simulink model "HMAUVSimulinkmobina"  (R2022b)
settings: Solver=ode45  StartTime=0.0  StopTime=80  MaxStep=0.01  RelTol=1e-3
libraries: slpidlib x6
settings Model: Creator=mobin  LastModifiedBy=mobin
settings SolverCC: AlgebraicLoopSolver=TrustRegion
settings DebuggingCC: UnconnectedInputMsg=warning  UnconnectedOutputMsg=warning  UnconnectedLineMsg=warning  SFMachineParentedDataDiag=warning
settings ModelReferenceCC: EnableRefExpFcnMdlSchedulingChecks=on
settings RTWCC: DLArmComputeVersion=19.05

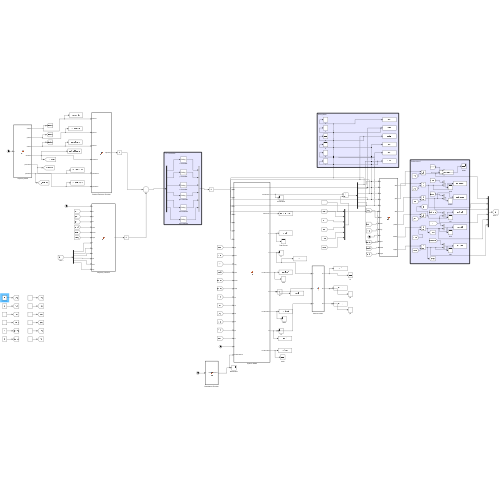
[thumbnail: Simulink's stored preview of the top-level diagram]
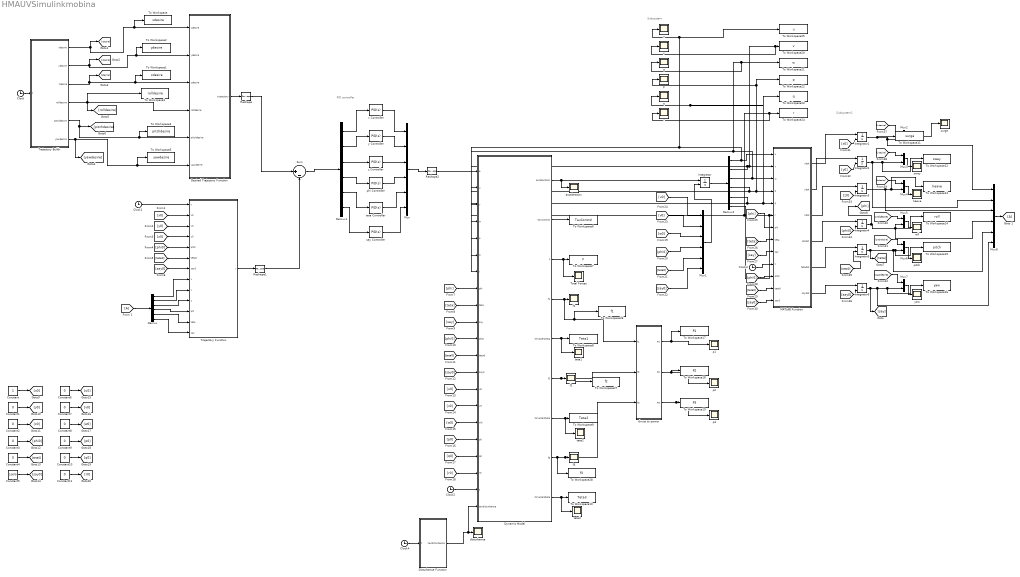
== system HMAUVSimulinkmobina ==
  note: Subsystem
  note: Subsystem1
  note: PID controller
  Clock{,1..4} (5 alike) : Clock
  Constant : Constant
  Constant{1..4,6..11} (10 alike) : Constant  Value=0
  Constant5 : Constant  Value=3.0079
  Demux : Demux  Outputs=6
  Demux1 : Demux  Outputs=6
  Demux2 : Demux  Outputs=6
  Desired Trajectory Function : MATLAB Function  TreatAsAtomicUnit=on
  Disturbance Function : MATLAB Function  TreatAsAtomicUnit=on
  Dynamic Model : MATLAB Function  TreatAsAtomicUnit=on
  From 1 : From
  Goto 1 : Goto
  Integrator{,1..6} (7 alike) : Integrator  InitialConditionSource=external
  MATLAB Function : MATLAB Function  TreatAsAtomicUnit=on
  Mux : Mux  Inputs=6
  Mux1 : Mux  Inputs=6
  Mux{2..7} (6 alike) : Mux  Inputs=2
  Mux8 : Mux  Inputs=6
  Reshape : Reshape  OutputDimensionality=Customize  OutputDimensions=[6,1]
  Reshape1 : Reshape  OutputDimensionality=Customize  OutputDimensions=[6,1]
  Reshape2 : Reshape  OutputDimensionality=Customize  OutputDimensions=[6,1]
  Sum : Sum  Inputs=|+-
  To Workspace : ToWorkspace  VariableName=xdesire  SaveFormat=Timeseries  SampleTime=-1
  To Workspace1 : ToWorkspace  VariableName=zdesire  SaveFormat=Timeseries  SampleTime=-1
  To Workspace10 : ToWorkspace  VariableName=Teta3  SaveFormat=Timeseries  SampleTime=-1
  To Workspace11 : ToWorkspace  VariableName=surge  SaveFormat=Timeseries  SampleTime=-1
  To Workspace12 : ToWorkspace  VariableName=sway  SaveFormat=Timeseries  SampleTime=-1
  To Workspace13 : ToWorkspace  VariableName=heave  SaveFormat=Timeseries  SampleTime=-1
  To Workspace14 : ToWorkspace  VariableName=roll  SaveFormat=Timeseries  SampleTime=-1
  To Workspace15 : ToWorkspace  VariableName=pitch  SaveFormat=Timeseries  SampleTime=-1
  To Workspace16 : ToWorkspace  VariableName=yaw  SaveFormat=Timeseries  SampleTime=-1
  To Workspace17 : ToWorkspace  VariableName=P1  SaveFormat=Timeseries  SampleTime=-1
  To Workspace18 : ToWorkspace  VariableName=P2  SaveFormat=Timeseries  SampleTime=-1
  To Workspace19 : ToWorkspace  VariableName=P3  SaveFormat=Timeseries  SampleTime=-1
  To Workspace2 : ToWorkspace  VariableName=ydesire  SaveFormat=Timeseries  SampleTime=-1
  To Workspace20 : ToWorkspace  VariableName=v  SaveFormat=Timeseries  SampleTime=-1
  To Workspace21 : ToWorkspace  VariableName=w  SaveFormat=Timeseries  SampleTime=-1
  To Workspace22 : ToWorkspace  VariableName=p  SaveFormat=Timeseries  SampleTime=-1
  To Workspace23 : ToWorkspace  VariableName=q  SaveFormat=Timeseries  SampleTime=-1
  To Workspace24 : ToWorkspace  VariableName=r  SaveFormat=Timeseries  SampleTime=-1
  To Workspace25 : ToWorkspace  VariableName=u  SaveFormat=Timeseries  SampleTime=-1
  To Workspace26 : ToWorkspace  VariableName=f1  SaveFormat=Timeseries  SampleTime=-1
  To Workspace27 : ToWorkspace  VariableName=f2  SaveFormat=Timeseries  SampleTime=-1
  To Workspace28 : ToWorkspace  VariableName=f3  SaveFormat=Timeseries  SampleTime=-1
  To Workspace3 : ToWorkspace  VariableName=rolldesire  SaveFormat=Timeseries  SampleTime=-1
  To Workspace4 : ToWorkspace  VariableName=pitchdesire  SaveFormat=Timeseries  SampleTime=-1
  To Workspace5 : ToWorkspace  VariableName=yawdesire  SaveFormat=Timeseries  SampleTime=-1
  To Workspace6 : ToWorkspace  VariableName=TavControl  SaveFormat=Timeseries  SampleTime=-1
  To Workspace7 : ToWorkspace  VariableName=F  SaveFormat=Timeseries  SampleTime=-1
  To Workspace8 : ToWorkspace  VariableName=Teta1  SaveFormat=Timeseries  SampleTime=-1
  To Workspace9 : ToWorkspace  VariableName=Teta2  SaveFormat=Timeseries  SampleTime=-1
  Total Forces : Scope
  Trajectory Buildr : MATLAB Function  TreatAsAtomicUnit=on
  Trajectory Function : MATLAB Function  TreatAsAtomicUnit=on
  acceleration : Scope
  disturbance : Scope
  f1 : Scope
  f2 : Scope
  f3 : Scope
  heave : Scope
  p{,1..3} (4 alike) : Scope
  phi Controller : slpidlib/PID Controller  Controller=PID  Form=Parallel  TimeDomain=Continuous-time  UseExternalTs=off  SampleTime=-1  IntegratorMethod=Forward Euler  FilterMethod=Forward Euler  ControllerParametersSource=internal  P=6000  I=0  UseKiTs=off  D=3000  N=100  UseFilter=on  TunerSelectOption=Transfer Function Based (PID Tuner App)  InitialConditionSource=internal  InitialConditionForIntegrator=0  InitialConditionForFilter=0  DifferentiatorICPrevScaledInput=0  ExternalReset=none  TrackingMode=off  Kt=1  LimitOutput=off  SatLimitsSource=internal  UpperSaturationLimit=inf  LowerSaturationLimit=-inf  LinearizeAsGain=on  AntiWindupMode=none  Kb=1  LimitIntegrator=off  UpperIntegratorSaturationLimit=inf  LowerIntegratorSaturationLimit=-inf  POutMin=[]  POutMax=[]  IOutMin=[]  IOutMax=[]  DOutMin=[]  DOutMax=[]  NOutMin=[]  NOutMax=[]  SumOutMin=[]  SumOutMax=[]  SaturationOutMin=[]  SaturationOutMax=[]  PParamMin=[]  PParamMax=[]  IParamMin=[]  IParamMax=[]  DParamMin=[]  DParamMax=[]  NParamMin=[]  NParamMax=[]  KbParamMin=[]  KbParamMax=[]  KtParamMin=[]  KtParamMax=[]  KbOutMin=[]  KbOutMax=[]  KtOutMin=[]  KtOutMax=[]  IntegratorOutMin=[]  IntegratorOutMax=[]  FilterOutMin=[]  FilterOutMax=[]  SumI1OutMin=[]  SumI1OutMax=[]  SumI2OutMin=[]  SumI2OutMax=[]  SumI3OutMin=[]  SumI3OutMax=[]  SumI4OutMin=[]  SumI4OutMax=[]  SumDOutMin=[]  SumDOutMax=[]  DifferentiatorOutMin=[]  DifferentiatorOutMax=[]  FilterDiffOutCoefMin=[]  FilterDiffOutCoefMax=[]  ReciprocalOutMin=[]  ReciprocalOutMax=[]  SumDenOutMin=[]  SumDenOutMax=[]  SumNumOutMin=[]  SumNumOutMax=[]  DivideOutMin=[]  DivideOutMax=[]  UdiffTsProdOutMin=[]  UdiffTsProdOutMax=[]  NTsProdOutMin=[]  NTsProdOutMax=[]  UintegralTsProdOutMin=[]  UintegralTsProdOutMax=[]  UngainTsProdOutMin=[]  UngainTsProdOutMax=[]  ClampingZeroOutDataTypeStr=Inherit: Inherit via back propagation  ClampingZeroOutMin=[]  ClampingZeroOutMax=[]  FilterDenConstantOutDataTypeStr=Inherit: Inherit via back propagation  FilterDenConstantOutMin=[]  FilterDenConstantOutMax=[]  PCopyOutDataTypeStr=Inherit: Inherit via back propagation  PCopyOutMin=[]  PCopyOutMax=[]  NCopyOutDataTypeStr=Inherit: Inherit via back propagation  NCopyOutMin=[]  NCopyOutMax=[]  IntegratorContinuousStateAttributes=''  IntegratorStateMustResolveToSignalObject=off  IntegratorRTWStateStorageClass=Auto  FilterContinuousStateAttributes=''  FilterStateMustResolveToSignalObject=off  FilterRTWStateStorageClass=Auto  ParallelPVariant=InternalParameters  IdealPVariant=Disabled  IVariant=InternalParameters  DVariant=InternalParameters  IntegratorVariant=Continuous  SatVariant=Disabled  AWVariant=Passthrough  PCopyVariant=Disabled  TRVariant=Disabled  FdbkBlocksVariant=Forward  IdealPFdbkVariant=Disabled  SatFdbkVariant=Disabled  DerivativeFilterVariant=ContFilter  NVariant=InternalParameters  NCopyVariant=Disabled  FilterICVariant=InternalICsFilter  IntegratorICVariant=InternalICs  ExternalResetVariant=Disabled  TRSumVariant=Passthrough  SumFdbkVariant=Disabled  SumVariant=Sum_PID  TsampFilterVariant=InternalTs  TsampNgainVariant=Passthrough  TsampIntegralVariant=Passthrough  ExternalSaturationOutDataTypeStr=Inherit: Same as second input
  pitch : Scope
  q : Scope
  r : Scope
  roll : Scope
  say Controller : slpidlib/PID Controller  Controller=PID  Form=Parallel  TimeDomain=Continuous-time  UseExternalTs=off  SampleTime=-1  IntegratorMethod=Forward Euler  FilterMethod=Forward Euler  ControllerParametersSource=internal  P=6000  I=0  UseKiTs=off  D=3000  N=100  UseFilter=on  TunerSelectOption=Transfer Function Based (PID Tuner App)  InitialConditionSource=internal  InitialConditionForIntegrator=0  InitialConditionForFilter=0  DifferentiatorICPrevScaledInput=0  ExternalReset=none  TrackingMode=off  Kt=1  LimitOutput=off  SatLimitsSource=internal  UpperSaturationLimit=inf  LowerSaturationLimit=-inf  LinearizeAsGain=on  AntiWindupMode=none  Kb=1  LimitIntegrator=off  UpperIntegratorSaturationLimit=inf  LowerIntegratorSaturationLimit=-inf  POutMin=[]  POutMax=[]  IOutMin=[]  IOutMax=[]  DOutMin=[]  DOutMax=[]  NOutMin=[]  NOutMax=[]  SumOutMin=[]  SumOutMax=[]  SaturationOutMin=[]  SaturationOutMax=[]  PParamMin=[]  PParamMax=[]  IParamMin=[]  IParamMax=[]  DParamMin=[]  DParamMax=[]  NParamMin=[]  NParamMax=[]  KbParamMin=[]  KbParamMax=[]  KtParamMin=[]  KtParamMax=[]  KbOutMin=[]  KbOutMax=[]  KtOutMin=[]  KtOutMax=[]  IntegratorOutMin=[]  IntegratorOutMax=[]  FilterOutMin=[]  FilterOutMax=[]  SumI1OutMin=[]  SumI1OutMax=[]  SumI2OutMin=[]  SumI2OutMax=[]  SumI3OutMin=[]  SumI3OutMax=[]  SumI4OutMin=[]  SumI4OutMax=[]  SumDOutMin=[]  SumDOutMax=[]  DifferentiatorOutMin=[]  DifferentiatorOutMax=[]  FilterDiffOutCoefMin=[]  FilterDiffOutCoefMax=[]  ReciprocalOutMin=[]  ReciprocalOutMax=[]  SumDenOutMin=[]  SumDenOutMax=[]  SumNumOutMin=[]  SumNumOutMax=[]  DivideOutMin=[]  DivideOutMax=[]  UdiffTsProdOutMin=[]  UdiffTsProdOutMax=[]  NTsProdOutMin=[]  NTsProdOutMax=[]  UintegralTsProdOutMin=[]  UintegralTsProdOutMax=[]  UngainTsProdOutMin=[]  UngainTsProdOutMax=[]  ClampingZeroOutDataTypeStr=Inherit: Inherit via back propagation  ClampingZeroOutMin=[]  ClampingZeroOutMax=[]  FilterDenConstantOutDataTypeStr=Inherit: Inherit via back propagation  FilterDenConstantOutMin=[]  FilterDenConstantOutMax=[]  PCopyOutDataTypeStr=Inherit: Inherit via back propagation  PCopyOutMin=[]  PCopyOutMax=[]  NCopyOutDataTypeStr=Inherit: Inherit via back propagation  NCopyOutMin=[]  NCopyOutMax=[]  IntegratorContinuousStateAttributes=''  IntegratorStateMustResolveToSignalObject=off  IntegratorRTWStateStorageClass=Auto  FilterContinuousStateAttributes=''  FilterStateMustResolveToSignalObject=off  FilterRTWStateStorageClass=Auto  ParallelPVariant=InternalParameters  IdealPVariant=Disabled  IVariant=InternalParameters  DVariant=InternalParameters  IntegratorVariant=Continuous  SatVariant=Disabled  AWVariant=Passthrough  PCopyVariant=Disabled  TRVariant=Disabled  FdbkBlocksVariant=Forward  IdealPFdbkVariant=Disabled  SatFdbkVariant=Disabled  DerivativeFilterVariant=ContFilter  NVariant=InternalParameters  NCopyVariant=Disabled  FilterICVariant=InternalICsFilter  IntegratorICVariant=InternalICs  ExternalResetVariant=Disabled  TRSumVariant=Passthrough  SumFdbkVariant=Disabled  SumVariant=Sum_PID  TsampFilterVariant=InternalTs  TsampNgainVariant=Passthrough  TsampIntegralVariant=Passthrough  ExternalSaturationOutDataTypeStr=Inherit: Same as second input
  surge : Scope
  sway : Scope
  teta Controller : slpidlib/PID Controller  Controller=PID  Form=Parallel  TimeDomain=Continuous-time  UseExternalTs=off  SampleTime=-1  IntegratorMethod=Forward Euler  FilterMethod=Forward Euler  ControllerParametersSource=internal  P=6000  I=0  UseKiTs=off  D=3000  N=100  UseFilter=on  TunerSelectOption=Transfer Function Based (PID Tuner App)  InitialConditionSource=internal  InitialConditionForIntegrator=0  InitialConditionForFilter=0  DifferentiatorICPrevScaledInput=0  ExternalReset=none  TrackingMode=off  Kt=1  LimitOutput=off  SatLimitsSource=internal  UpperSaturationLimit=inf  LowerSaturationLimit=-inf  LinearizeAsGain=on  AntiWindupMode=none  Kb=1  LimitIntegrator=off  UpperIntegratorSaturationLimit=inf  LowerIntegratorSaturationLimit=-inf  POutMin=[]  POutMax=[]  IOutMin=[]  IOutMax=[]  DOutMin=[]  DOutMax=[]  NOutMin=[]  NOutMax=[]  SumOutMin=[]  SumOutMax=[]  SaturationOutMin=[]  SaturationOutMax=[]  PParamMin=[]  PParamMax=[]  IParamMin=[]  IParamMax=[]  DParamMin=[]  DParamMax=[]  NParamMin=[]  NParamMax=[]  KbParamMin=[]  KbParamMax=[]  KtParamMin=[]  KtParamMax=[]  KbOutMin=[]  KbOutMax=[]  KtOutMin=[]  KtOutMax=[]  IntegratorOutMin=[]  IntegratorOutMax=[]  FilterOutMin=[]  FilterOutMax=[]  SumI1OutMin=[]  SumI1OutMax=[]  SumI2OutMin=[]  SumI2OutMax=[]  SumI3OutMin=[]  SumI3OutMax=[]  SumI4OutMin=[]  SumI4OutMax=[]  SumDOutMin=[]  SumDOutMax=[]  DifferentiatorOutMin=[]  DifferentiatorOutMax=[]  FilterDiffOutCoefMin=[]  FilterDiffOutCoefMax=[]  ReciprocalOutMin=[]  ReciprocalOutMax=[]  SumDenOutMin=[]  SumDenOutMax=[]  SumNumOutMin=[]  SumNumOutMax=[]  DivideOutMin=[]  DivideOutMax=[]  UdiffTsProdOutMin=[]  UdiffTsProdOutMax=[]  NTsProdOutMin=[]  NTsProdOutMax=[]  UintegralTsProdOutMin=[]  UintegralTsProdOutMax=[]  UngainTsProdOutMin=[]  UngainTsProdOutMax=[]  ClampingZeroOutDataTypeStr=Inherit: Inherit via back propagation  ClampingZeroOutMin=[]  ClampingZeroOutMax=[]  FilterDenConstantOutDataTypeStr=Inherit: Inherit via back propagation  FilterDenConstantOutMin=[]  FilterDenConstantOutMax=[]  PCopyOutDataTypeStr=Inherit: Inherit via back propagation  PCopyOutMin=[]  PCopyOutMax=[]  NCopyOutDataTypeStr=Inherit: Inherit via back propagation  NCopyOutMin=[]  NCopyOutMax=[]  IntegratorContinuousStateAttributes=''  IntegratorStateMustResolveToSignalObject=off  IntegratorRTWStateStorageClass=Auto  FilterContinuousStateAttributes=''  FilterStateMustResolveToSignalObject=off  FilterRTWStateStorageClass=Auto  ParallelPVariant=InternalParameters  IdealPVariant=Disabled  IVariant=InternalParameters  DVariant=InternalParameters  IntegratorVariant=Continuous  SatVariant=Disabled  AWVariant=Passthrough  PCopyVariant=Disabled  TRVariant=Disabled  FdbkBlocksVariant=Forward  IdealPFdbkVariant=Disabled  SatFdbkVariant=Disabled  DerivativeFilterVariant=ContFilter  NVariant=InternalParameters  NCopyVariant=Disabled  FilterICVariant=InternalICsFilter  IntegratorICVariant=InternalICs  ExternalResetVariant=Disabled  TRSumVariant=Passthrough  SumFdbkVariant=Disabled  SumVariant=Sum_PID  TsampFilterVariant=InternalTs  TsampNgainVariant=Passthrough  TsampIntegralVariant=Passthrough  ExternalSaturationOutDataTypeStr=Inherit: Same as second input
  teta1 : Scope
  teta2 : Scope
  teta3 : Scope
  thrust to power : MATLAB Function  TreatAsAtomicUnit=on
  u : Scope
  v : Scope
  w : Scope
  x Controller : slpidlib/PID Controller  Controller=PID  Form=Parallel  TimeDomain=Continuous-time  UseExternalTs=off  SampleTime=-1  IntegratorMethod=Forward Euler  FilterMethod=Forward Euler  ControllerParametersSource=internal  P=6000  I=0  UseKiTs=off  D=3000  N=100  UseFilter=on  TunerSelectOption=Transfer Function Based (PID Tuner App)  InitialConditionSource=internal  InitialConditionForIntegrator=0  InitialConditionForFilter=0  DifferentiatorICPrevScaledInput=0  ExternalReset=none  TrackingMode=off  Kt=1  LimitOutput=off  SatLimitsSource=internal  UpperSaturationLimit=inf  LowerSaturationLimit=-inf  LinearizeAsGain=on  AntiWindupMode=none  Kb=1  LimitIntegrator=off  UpperIntegratorSaturationLimit=inf  LowerIntegratorSaturationLimit=-inf  POutMin=[]  POutMax=[]  IOutMin=[]  IOutMax=[]  DOutMin=[]  DOutMax=[]  NOutMin=[]  NOutMax=[]  SumOutMin=[]  SumOutMax=[]  SaturationOutMin=[]  SaturationOutMax=[]  PParamMin=[]  PParamMax=[]  IParamMin=[]  IParamMax=[]  DParamMin=[]  DParamMax=[]  NParamMin=[]  NParamMax=[]  KbParamMin=[]  KbParamMax=[]  KtParamMin=[]  KtParamMax=[]  KbOutMin=[]  KbOutMax=[]  KtOutMin=[]  KtOutMax=[]  IntegratorOutMin=[]  IntegratorOutMax=[]  FilterOutMin=[]  FilterOutMax=[]  SumI1OutMin=[]  SumI1OutMax=[]  SumI2OutMin=[]  SumI2OutMax=[]  SumI3OutMin=[]  SumI3OutMax=[]  SumI4OutMin=[]  SumI4OutMax=[]  SumDOutMin=[]  SumDOutMax=[]  DifferentiatorOutMin=[]  DifferentiatorOutMax=[]  FilterDiffOutCoefMin=[]  FilterDiffOutCoefMax=[]  ReciprocalOutMin=[]  ReciprocalOutMax=[]  SumDenOutMin=[]  SumDenOutMax=[]  SumNumOutMin=[]  SumNumOutMax=[]  DivideOutMin=[]  DivideOutMax=[]  UdiffTsProdOutMin=[]  UdiffTsProdOutMax=[]  NTsProdOutMin=[]  NTsProdOutMax=[]  UintegralTsProdOutMin=[]  UintegralTsProdOutMax=[]  UngainTsProdOutMin=[]  UngainTsProdOutMax=[]  ClampingZeroOutDataTypeStr=Inherit: Inherit via back propagation  ClampingZeroOutMin=[]  ClampingZeroOutMax=[]  FilterDenConstantOutDataTypeStr=Inherit: Inherit via back propagation  FilterDenConstantOutMin=[]  FilterDenConstantOutMax=[]  PCopyOutDataTypeStr=Inherit: Inherit via back propagation  PCopyOutMin=[]  PCopyOutMax=[]  NCopyOutDataTypeStr=Inherit: Inherit via back propagation  NCopyOutMin=[]  NCopyOutMax=[]  IntegratorContinuousStateAttributes=''  IntegratorStateMustResolveToSignalObject=off  IntegratorRTWStateStorageClass=Auto  FilterContinuousStateAttributes=''  FilterStateMustResolveToSignalObject=off  FilterRTWStateStorageClass=Auto  ParallelPVariant=InternalParameters  IdealPVariant=Disabled  IVariant=InternalParameters  DVariant=InternalParameters  IntegratorVariant=Continuous  SatVariant=Disabled  AWVariant=Passthrough  PCopyVariant=Disabled  TRVariant=Disabled  FdbkBlocksVariant=Forward  IdealPFdbkVariant=Disabled  SatFdbkVariant=Disabled  DerivativeFilterVariant=ContFilter  NVariant=InternalParameters  NCopyVariant=Disabled  FilterICVariant=InternalICsFilter  IntegratorICVariant=InternalICs  ExternalResetVariant=Disabled  TRSumVariant=Passthrough  SumFdbkVariant=Disabled  SumVariant=Sum_PID  TsampFilterVariant=InternalTs  TsampNgainVariant=Passthrough  TsampIntegralVariant=Passthrough  ExternalSaturationOutDataTypeStr=Inherit: Same as second input
  y Controller : slpidlib/PID Controller  Controller=PID  Form=Parallel  TimeDomain=Continuous-time  UseExternalTs=off  SampleTime=-1  IntegratorMethod=Forward Euler  FilterMethod=Forward Euler  ControllerParametersSource=internal  P=6000  I=0  UseKiTs=off  D=3000  N=100  UseFilter=on  TunerSelectOption=Transfer Function Based (PID Tuner App)  InitialConditionSource=internal  InitialConditionForIntegrator=0  InitialConditionForFilter=0  DifferentiatorICPrevScaledInput=0  ExternalReset=none  TrackingMode=off  Kt=1  LimitOutput=off  SatLimitsSource=internal  UpperSaturationLimit=inf  LowerSaturationLimit=-inf  LinearizeAsGain=on  AntiWindupMode=none  Kb=1  LimitIntegrator=off  UpperIntegratorSaturationLimit=inf  LowerIntegratorSaturationLimit=-inf  POutMin=[]  POutMax=[]  IOutMin=[]  IOutMax=[]  DOutMin=[]  DOutMax=[]  NOutMin=[]  NOutMax=[]  SumOutMin=[]  SumOutMax=[]  SaturationOutMin=[]  SaturationOutMax=[]  PParamMin=[]  PParamMax=[]  IParamMin=[]  IParamMax=[]  DParamMin=[]  DParamMax=[]  NParamMin=[]  NParamMax=[]  KbParamMin=[]  KbParamMax=[]  KtParamMin=[]  KtParamMax=[]  KbOutMin=[]  KbOutMax=[]  KtOutMin=[]  KtOutMax=[]  IntegratorOutMin=[]  IntegratorOutMax=[]  FilterOutMin=[]  FilterOutMax=[]  SumI1OutMin=[]  SumI1OutMax=[]  SumI2OutMin=[]  SumI2OutMax=[]  SumI3OutMin=[]  SumI3OutMax=[]  SumI4OutMin=[]  SumI4OutMax=[]  SumDOutMin=[]  SumDOutMax=[]  DifferentiatorOutMin=[]  DifferentiatorOutMax=[]  FilterDiffOutCoefMin=[]  FilterDiffOutCoefMax=[]  ReciprocalOutMin=[]  ReciprocalOutMax=[]  SumDenOutMin=[]  SumDenOutMax=[]  SumNumOutMin=[]  SumNumOutMax=[]  DivideOutMin=[]  DivideOutMax=[]  UdiffTsProdOutMin=[]  UdiffTsProdOutMax=[]  NTsProdOutMin=[]  NTsProdOutMax=[]  UintegralTsProdOutMin=[]  UintegralTsProdOutMax=[]  UngainTsProdOutMin=[]  UngainTsProdOutMax=[]  ClampingZeroOutDataTypeStr=Inherit: Inherit via back propagation  ClampingZeroOutMin=[]  ClampingZeroOutMax=[]  FilterDenConstantOutDataTypeStr=Inherit: Inherit via back propagation  FilterDenConstantOutMin=[]  FilterDenConstantOutMax=[]  PCopyOutDataTypeStr=Inherit: Inherit via back propagation  PCopyOutMin=[]  PCopyOutMax=[]  NCopyOutDataTypeStr=Inherit: Inherit via back propagation  NCopyOutMin=[]  NCopyOutMax=[]  IntegratorContinuousStateAttributes=''  IntegratorStateMustResolveToSignalObject=off  IntegratorRTWStateStorageClass=Auto  FilterContinuousStateAttributes=''  FilterStateMustResolveToSignalObject=off  FilterRTWStateStorageClass=Auto  ParallelPVariant=InternalParameters  IdealPVariant=Disabled  IVariant=InternalParameters  DVariant=InternalParameters  IntegratorVariant=Continuous  SatVariant=Disabled  AWVariant=Passthrough  PCopyVariant=Disabled  TRVariant=Disabled  FdbkBlocksVariant=Forward  IdealPFdbkVariant=Disabled  SatFdbkVariant=Disabled  DerivativeFilterVariant=ContFilter  NVariant=InternalParameters  NCopyVariant=Disabled  FilterICVariant=InternalICsFilter  IntegratorICVariant=InternalICs  ExternalResetVariant=Disabled  TRSumVariant=Passthrough  SumFdbkVariant=Disabled  SumVariant=Sum_PID  TsampFilterVariant=InternalTs  TsampNgainVariant=Passthrough  TsampIntegralVariant=Passthrough  ExternalSaturationOutDataTypeStr=Inherit: Same as second input
  yaw : Scope
  z Controller : slpidlib/PID Controller  Controller=PID  Form=Parallel  TimeDomain=Continuous-time  UseExternalTs=off  SampleTime=-1  IntegratorMethod=Forward Euler  FilterMethod=Forward Euler  ControllerParametersSource=internal  P=6000  I=0  UseKiTs=off  D=3000  N=100  UseFilter=on  TunerSelectOption=Transfer Function Based (PID Tuner App)  InitialConditionSource=internal  InitialConditionForIntegrator=0  InitialConditionForFilter=0  DifferentiatorICPrevScaledInput=0  ExternalReset=none  TrackingMode=off  Kt=1  LimitOutput=off  SatLimitsSource=internal  UpperSaturationLimit=inf  LowerSaturationLimit=-inf  LinearizeAsGain=on  AntiWindupMode=none  Kb=1  LimitIntegrator=off  UpperIntegratorSaturationLimit=inf  LowerIntegratorSaturationLimit=-inf  POutMin=[]  POutMax=[]  IOutMin=[]  IOutMax=[]  DOutMin=[]  DOutMax=[]  NOutMin=[]  NOutMax=[]  SumOutMin=[]  SumOutMax=[]  SaturationOutMin=[]  SaturationOutMax=[]  PParamMin=[]  PParamMax=[]  IParamMin=[]  IParamMax=[]  DParamMin=[]  DParamMax=[]  NParamMin=[]  NParamMax=[]  KbParamMin=[]  KbParamMax=[]  KtParamMin=[]  KtParamMax=[]  KbOutMin=[]  KbOutMax=[]  KtOutMin=[]  KtOutMax=[]  IntegratorOutMin=[]  IntegratorOutMax=[]  FilterOutMin=[]  FilterOutMax=[]  SumI1OutMin=[]  SumI1OutMax=[]  SumI2OutMin=[]  SumI2OutMax=[]  SumI3OutMin=[]  SumI3OutMax=[]  SumI4OutMin=[]  SumI4OutMax=[]  SumDOutMin=[]  SumDOutMax=[]  DifferentiatorOutMin=[]  DifferentiatorOutMax=[]  FilterDiffOutCoefMin=[]  FilterDiffOutCoefMax=[]  ReciprocalOutMin=[]  ReciprocalOutMax=[]  SumDenOutMin=[]  SumDenOutMax=[]  SumNumOutMin=[]  SumNumOutMax=[]  DivideOutMin=[]  DivideOutMax=[]  UdiffTsProdOutMin=[]  UdiffTsProdOutMax=[]  NTsProdOutMin=[]  NTsProdOutMax=[]  UintegralTsProdOutMin=[]  UintegralTsProdOutMax=[]  UngainTsProdOutMin=[]  UngainTsProdOutMax=[]  ClampingZeroOutDataTypeStr=Inherit: Inherit via back propagation  ClampingZeroOutMin=[]  ClampingZeroOutMax=[]  FilterDenConstantOutDataTypeStr=Inherit: Inherit via back propagation  FilterDenConstantOutMin=[]  FilterDenConstantOutMax=[]  PCopyOutDataTypeStr=Inherit: Inherit via back propagation  PCopyOutMin=[]  PCopyOutMax=[]  NCopyOutDataTypeStr=Inherit: Inherit via back propagation  NCopyOutMin=[]  NCopyOutMax=[]  IntegratorContinuousStateAttributes=''  IntegratorStateMustResolveToSignalObject=off  IntegratorRTWStateStorageClass=Auto  FilterContinuousStateAttributes=''  FilterStateMustResolveToSignalObject=off  FilterRTWStateStorageClass=Auto  ParallelPVariant=InternalParameters  IdealPVariant=Disabled  IVariant=InternalParameters  DVariant=InternalParameters  IntegratorVariant=Continuous  SatVariant=Disabled  AWVariant=Passthrough  PCopyVariant=Disabled  TRVariant=Disabled  FdbkBlocksVariant=Forward  IdealPFdbkVariant=Disabled  SatFdbkVariant=Disabled  DerivativeFilterVariant=ContFilter  NVariant=InternalParameters  NCopyVariant=Disabled  FilterICVariant=InternalICsFilter  IntegratorICVariant=InternalICs  ExternalResetVariant=Disabled  TRSumVariant=Passthrough  SumFdbkVariant=Disabled  SumVariant=Sum_PID  TsampFilterVariant=InternalTs  TsampNgainVariant=Passthrough  TsampIntegralVariant=Passthrough  ExternalSaturationOutDataTypeStr=Inherit: Same as second input
  wires:
  Clock/1 -> Trajectory Buildr/1(t)
  Trajectory Buildr/1(xdesire) -> To Workspace/1, Desired Trajectory Function/1(xdesire), [xdesire]
  Trajectory Buildr/2(ydesire) -> To Workspace2/1, Desired Trajectory Function/2(ydesire), [ydesire]
  Trajectory Buildr/3(zdesire) -> [zdesire], To Workspace1/1, Desired Trajectory Function/3(zdesire)
  Clock1/1 -> Trajectory Function/1(t)
  Demux/1 -> Trajectory Function/8(x)
  Demux/2 -> Trajectory Function/9(y)
  Demux/3 -> Trajectory Function/10(z)
  Demux/4 -> Trajectory Function/11(phi)
  Demux/5 -> Trajectory Function/12(teta)
  Demux/6 -> Trajectory Function/13(say)
  From 1/1 -> Demux/1
  [x0] -> Trajectory Function/2(x0)
  [y0] -> Trajectory Function/3(y0)
  [z0] -> Trajectory Function/4(z0)
  [phi0] -> Trajectory Function/5(phi0)
  [teta0] -> Trajectory Function/6(teta0)
  [say0] -> Trajectory Function/7(say0)
  Trajectory Function/1(r) -> Reshape1/1
  Desired Trajectory Function/1(trajectory) -> Reshape/1
  [phi] -> Dynamic Model/8(phi)
  [teta] -> Dynamic Model/9(teta)
  [say] -> Dynamic Model/10(say)
  [phi0] -> Dynamic Model/11(phi0)
  [teta0] -> Dynamic Model/12(teta0)
  [say0] -> Dynamic Model/13(say0)
  [u0] -> Dynamic Model/14(u0)
  [v0] -> Dynamic Model/15(v0)
  [w0] -> Dynamic Model/16(w0)
  [p0] -> Dynamic Model/17(p0)
  [q0] -> Dynamic Model/18(q0)
  [r0] -> Dynamic Model/19(r0)
  Clock2/1 -> Dynamic Model/20(t)
  Dynamic Model/3(F) -> Total Forces/1, To Workspace7/1
  Dynamic Model/5(thruster1teta) -> teta1/1, To Workspace8/1
  Dynamic Model/7(thruster2teta) -> teta2/1, To Workspace9/1
  Dynamic Model/9(thruster3teta) -> teta3/1, To Workspace10/1
  Dynamic Model/4(f1) -> To Workspace26/1, thrust to power/1(f1), f1/1
  Dynamic Model/6(f2) -> To Workspace27/1, thrust to power/2(f2), f2/1
  Dynamic Model/8(f3) -> To Workspace28/1, thrust to power/3(f3), f3/1
  [u0] -> Mux1/1
  [v0] -> Mux1/2
  [w0] -> Mux1/3
  [phi0] -> Mux1/4
  [teta0] -> Mux1/5
  [say0] -> Mux1/6
  Mux1/1 -> Integrator/2
  Dynamic Model/1(accelaration) -> acceleration/1, Integrator/1
  Integrator/1 -> Demux2/1
  [phi] -> MATLAB Function/7(phi)
  [teta] -> MATLAB Function/8(teta)
  [say] -> MATLAB Function/9(say)
  [phi0] -> MATLAB Function/11(phi0)
  [teta0] -> MATLAB Function/12(teta0)
  [say0] -> MATLAB Function/13(say0)
  Clock3/1 -> MATLAB Function/10(t)
  Mux8/1 -> Goto 1/1
  thrust to power/1(P1) -> p1/1, To Workspace17/1
  thrust to power/2(P2) -> To Workspace18/1, p2/1
  thrust to power/3(P3) -> p3/1, To Workspace19/1
  Reshape/1 -> Sum/1
  Reshape1/1 -> Sum/2
  Constant/1 -> [x0]
  Constant1/1 -> [y0]
  Constant2/1 -> [z0]
  Constant3/1 -> [phi0]
  Constant4/1 -> [teta0]
  Constant5/1 -> [say0]
  Constant6/1 -> [u0]
  Constant7/1 -> [v0]
  Constant8/1 -> [w0]
  Constant9/1 -> [p0]
  Constant10/1 -> [q0]
  Constant11/1 -> [r0]
  Clock4/1 -> Disturbance Function/1(t)
  Disturbance Function/1(tavdisturbance) -> Dynamic Model/21(tavdisturbance), disturbance/1
  Reshape2/1 -> Dynamic Model/1(e)
  Mux/1 -> Reshape2/1
  Trajectory Buildr/4(rolldesire) -> Desired Trajectory Function/4(rolldesire), To Workspace3/1, [rolldesire]
  Trajectory Buildr/5(pitchdesire) -> [pitchdesire], To Workspace4/1, Desired Trajectory Function/5(pitchdesire)
  Trajectory Buildr/6(yawdesire) -> [yawdesire], To Workspace5/1, Desired Trajectory Function/6(yawdesire)
  Dynamic Model/2(TAVcontrol) -> To Workspace6/1
  Sum/1 -> Demux1/1
  phi Controller/1 -> Mux/4
  y Controller/1 -> Mux/2
  Demux1/3 -> z Controller/1
  Demux1/5 -> teta Controller/1
  x Controller/1 -> Mux/1
  Demux1/6 -> say Controller/1
  z Controller/1 -> Mux/3
  Demux1/1 -> x Controller/1
  Demux1/4 -> phi Controller/1
  say Controller/1 -> Mux/6
  Demux1/2 -> y Controller/1
  teta Controller/1 -> Mux/5
  Integrator1/1 -> To Workspace11/1, Mux8/1, Mux2/2
  Integrator2/1 -> Mux8/2, To Workspace12/1, Mux3/2
  Integrator3/1 -> Mux8/3, To Workspace13/1, Mux4/2
  Integrator4/1 -> [phi], Mux5/2, Mux8/4, To Workspace14/1
  Integrator5/1 -> [teta], Mux8/5, To Workspace15/1, Mux6/2
  Integrator6/1 -> [say], Mux8/6, To Workspace16/1, Mux7/2
  MATLAB Function/3(zdot) -> Integrator3/1
  MATLAB Function/6(saydot) -> Integrator6/1
  [xdesire] -> Mux2/1
  Mux5/1 -> roll/1
  Mux6/1 -> pitch/1
  MATLAB Function/4(phidot) -> Integrator4/1
  Mux2/1 -> surge/1
  MATLAB Function/1(xdot) -> Integrator1/1
  Mux3/1 -> sway/1
  MATLAB Function/5(tetadot) -> Integrator5/1
  Mux7/1 -> yaw/1
  [yawdesire] -> Mux7/1
  [phi0] -> Integrator4/2
  [pitchdesire] -> Mux6/1
  [say0] -> Integrator6/2
  [rolldesire] -> Mux5/1
  [ydesire] -> Mux3/1
  [y0] -> Integrator2/2
  Mux4/1 -> heave/1
  [teta0] -> Integrator5/2
  [z0] -> Integrator3/2
  [x0] -> Integrator1/2
  MATLAB Function/2(ydot) -> Integrator2/1
  [zdesire] -> Mux4/1
  Demux2/3 -> Dynamic Model/4(w), w/1, To Workspace21/1, MATLAB Function/3(w)
  Demux2/4 -> To Workspace22/1, p/1, MATLAB Function/4(p), Dynamic Model/5(p)
  Demux2/5 -> MATLAB Function/5(q), To Workspace23/1, q/1, Dynamic Model/6(q)
  Demux2/1 -> MATLAB Function/1(u), Dynamic Model/2(u), To Workspace25/1, u/1
  Demux2/6 -> r/1, To Workspace24/1, Dynamic Model/7(r), MATLAB Function/6(r)
  Demux2/2 -> v/1, To Workspace20/1, MATLAB Function/2(v), Dynamic Model/3(v)

== matlab function HMAUVSimulinkmobina/MATLAB Function ==
  data: u input; xdot output; v input; w input; p input; q input; r input; phi input; teta input; say input; t input; phi0 input; teta0 input; say0 input; ydot output; zdot output; phidot output; tetadot output; saydot output
function [xdot,ydot,zdot,phidot,tetadot,saydot] = fcn(u,v,w,p,q,r,phi,teta,say,t,phi0,teta0,say0)

%this block is to generate the current position of the vehicle

%using if statement for checking if it is the initial position or not
if t==0
    phi=phi0;
    teta=teta0;
    say=say0;
end

%for non initial positions, the transformation matrices will be used to
%transform from body to earth frame the corresponding velocities being
%calculated by integration of the acceleration
J1eta2=[cos(say)*cos(teta) , -sin(say)*cos(phi)+cos(say)*sin(teta)*sin(phi) ,sin(say)*sin(phi)+cos(say)*sin(teta)*cos(phi);sin(say)*cos(teta),cos(say)*cos(phi)+sin(say)*sin(teta)*sin(phi),-cos(say)*sin(phi)+sin(say)*sin(teta)*cos(phi);-sin(teta),cos(teta)*sin(phi),cos(teta)*cos(phi)];
J2eta2=[1,sin(phi)*tan(teta),cos(phi)*tan(teta);0,cos(phi),-sin(phi);0,sin(phi)/cos(teta),cos(phi)/cos(teta)];
Jeta=[ J1eta2 zeros(3,3);zeros(3,3) J2eta2 ];

xdot=Jeta(1,1)*u+Jeta(1,2)*v+Jeta(1,3)*w+Jeta(1,4)*p+Jeta(1,5)*q+Jeta(1,6)*r;
ydot=Jeta(2,1)*u+ Jeta(2,2)*v+ Jeta(2,3)*w+Jeta(2,4)*p+Jeta(2,5)*q+Jeta(2,6)*r;
zdot=Jeta(3,1)*u+Jeta(3,2)*v+Jeta(3,3)*w+ Jeta(3,4)*p+ Jeta(3,5)*q+Jeta(3,6)*r;
phidot=Jeta(4,1)*u+Jeta(4,2)*v+Jeta(4,3)*w+ Jeta(4,4)*p+ Jeta(4,5)*q+Jeta(4,6)*r;
tetadot=Jeta(5,1)*u+Jeta(5,2)*v+Jeta(5,3)*w+ Jeta(5,4)*p+ Jeta(5,5)*q+Jeta(5,6)*r;
saydot=Jeta(6,1)*u+Jeta(6,2)*v+ Jeta(6,3)*w+ Jeta(6,4)*p+Jeta(6,5)*q+Jeta(6,6)*r;

== matlab function HMAUVSimulinkmobina/thrust to power ==
  data: P1 output; f1 input; f2 input; f3 input; P2 output; P3 output
function [P1,P2,P3] = fcn(f1,f2,f3)

%the max produced thrust can be 28.4 N (based on thruster property)
if f1>28.4
    f1=28.4;
end
if f2>28.4
    f2=28.4;
end
if f3>28.4
    f3=28.4;
end

%the generated power for each thruster can be calculated by the equations
%from datasheet of the thruster company (unit W)

P1 = 0.2318*f1^2 + 0.52*f1 + 6.6267;
P2 = 0.2318*f2^2 + 0.52*f2 + 6.6267;
P3 = 0.2318*f3^2 + 0.52*f3 + 6.6267;

end

== matlab function HMAUVSimulinkmobina/Disturbance Function ==
  data: t input; tavdisturbance output
function tavdisturbance  = fcn(t)
%this is the disturbane function introduced to the vehicle, due to the
%limitations of the current controller (PID), it is set to be zero but it
%is a topic that can be further expanded for more complex controllers 
     tavdx=0;
    tavdy=0;
    tavdz=0;
    tavdmx=0;
    tavdmy=0;
    tavdmz=0;
if and(t>1,t<150)
    tavdx=0;
    tavdy=0;
    tavdz=0;
    tavdmx=0;
    tavdmy=0;
    tavdmz=0;
    

end
tavdisturbance=[tavdx;tavdy;tavdz; tavdmx;tavdmy;tavdmz];

== matlab function HMAUVSimulinkmobina/Desired Trajectory Function ==
  data: xdesire input; trajectory output; ydesire input; zdesire input; rolldesire input; pitchdesire input; yawdesire input
function trajectory  = fcn(xdesire,ydesire,zdesire,rolldesire,pitchdesire,yawdesire)

%the desired x, y, z, roll, pitch and yaw being introduced as a singular trajectory 
trajectory1=xdesire;
trajectory2=ydesire;
trajectory3=zdesire;
trajectory4=rolldesire;
trajectory5=pitchdesire;
trajectory6=yawdesire;
trajectory=[trajectory1;trajectory2;trajectory3;trajectory4;trajectory5;trajectory6];

== matlab function HMAUVSimulinkmobina/Trajectory Buildr ==
  data: t input; xdesire output; ydesire output; zdesire output; rolldesire output; pitchdesire output; yawdesire output
function [xdesire,ydesire,zdesire,rolldesire,pitchdesire,yawdesire] = fcn(t)

% this is the desired x, y, z, roll, pitch and yaw equations for spiral
% motion
w=pi/10;
xdesire=exp(-0.01*t)*cos(w*t);
ydesire=exp(-0.01*t)*sin(w*t);
zdesire=0.25*t;
rolldesire=pi*sin(w*t);
pitchdesire=(pi/3)*cos(w*t);
yawdesire=0.25*t;

% %for complex motion (viviani curve)
% R=1;
% w=pi/10;
% 
%  xdesire=2*R*cos(w*t/2)^2;
%  ydesire=2*R*sin(w*t/2)*cos(w*t/2);
%  zdesire=2*R*sin(w*t/2);
%  
%  rolldesire=(pi/2)*sin(w*t);
%  pitchdesire=(pi/3)*sin(w*t);
%  yawdesire=(pi/2)*sin(w*t);
 

end

== matlab function HMAUVSimulinkmobina/Trajectory Function ==
  data: t input; r output; x0 input; y0 input; z0 input; phi0 input; teta0 input; say0 input; x input; y input; z input; phi input; teta input; say input
function r = fcn(t,x0,y0,z0,phi0,teta0,say0,x,y,z,phi,teta,say)

%the functions to define the current location of the vehicle

%checking that if the vechicle is at the initial time, the vehicle is define to be at the place of initial
%parmeters x0, y0, z0, phi0, teta0, say0 otherwise at the current place
%being calculated in the future blocks
if t==0
    r=[x0; y0 ; z0; phi0; teta0; say0 ]
else
    r=[x ;y  ; z; phi ;teta ;say];
end

== matlab function HMAUVSimulinkmobina/Dynamic Model ==
  data: e input; u input; accelaration output; TAVcontrol output; v input; w input; p input; q input; r input; phi input; teta input; say input; phi0 input; teta0 input; say0 input; u0 input; v0 input; w0 input; p0 input; q0 input; r0 input; t input; F output; f1 output; thruster1teta output; f2 output; thruster2teta output; f3 output; thruster3teta output; tavdisturbance input
 function [accelaration,TAVcontrol,F,f1,thruster1teta,f2,thruster2teta,f3,thruster3teta]  = fcn(e,u,v,w,p,q,r,phi,teta,say,phi0,teta0,say0,u0,v0,w0,p0,q0,r0,t,tavdisturbance)

% setting everything to zero as the initial condition of the vehicle
fxthruster1=0;
fxthruster2=0;
fxthruster3=0;

fythruster1=0;
fythruster2=0;
fythruster3=0;

fzthruster1=0;
fzthruster2=0;
fzthruster3=0;

if t==0
    phi=phi0;
    teta=teta0;
    say=say0;
    u=u0;
    v=v0;
    w=w0;
    p=p0;
    q=q0;
    r=r0;
   
end

check=0;


%physical parameters of the vehicle (m)
%w=yl=yr;
width=0.45;
%l=xt+xl=xt+xr;
l=0.885;
m= 12.437;



%%Jacobian aka transformation Matrix for linear velovcity conversion from
%%earth to body frame
J1eta2=[cos(say)*cos(teta) , -sin(say)*cos(phi)+cos(say)*sin(teta)*sin(phi) ,sin(say)*sin(phi)+cos(say)*sin(teta)*cos(phi);sin(say)*cos(teta),cos(say)*cos(phi)+sin(say)*sin(teta)*sin(phi),-cos(say)*sin(phi)+sin(say)*sin(teta)*cos(phi);-sin(teta),cos(teta)*sin(phi),cos(teta)*cos(phi)];
%%Jacobian Matrix for angular velovcity conversionfrom earth to body frame
J2eta2=[1,sin(phi)*tan(teta),cos(phi)*tan(teta);0,cos(phi),-sin(phi);0,sin(phi)/cos(teta),cos(phi)/cos(teta)]
%%combining both of Jacobian matrices to one matrix 
Jeta=[ J1eta2 zeros(3,3);zeros(3,3) J2eta2 ]
%inverse of jeta matrix
Jinv=inv(Jeta)



%other physical parameters of the vehicle (m)
%xg=yr=yl;
xg=0.45;
%yg=xt;
yg=0.75;
zg=0.12;

%vehicle's inertial parameters (kgm^2)
Ixx=6741.44;
Ixy=1906.18;
Ixz=3580.59;
Iyx=1906.18;
Iyy=8454.36;
Iyz=2508.82;
Izx=3580.59;
Izy=2508.82;
Izz=4399.80;

%%hydrodynamic coefficients (to be defined by simulation, probably Ansys),
%%same data is being used as the work of Mr. Kadkhodaei. More work needs to
%%be done to gather data 
Xudot=-39.2
Xvdot=0;
Xwdot=0;
Xpdot=0;
Xqdot=0;
Xrdot=0;
Yudot=0;
Yvdot=-75.94;
Ywdot=0;
Ypdot=0;
Yqdot=0;
Yrdot=0;
Zudot=0;
Zvdot=0;
Zwdot=-111.47;
Zpdot=0;
Zqdot=0;
Zrdot=0;
Kudot=0;
Kvdot=0;
Kwdot=0;
Kpdot=-3.37;
Kqdot=0;
Krdot=0;
Mudot=0;
Mvdot=0;
Mwdot=0;
Mpdot=0;
Mqdot=-5.61;
Mrdot=0;
Nudot=0;
Nvdot=0;
Nwdot=0;
Npdot=0;
Nqdot=0;
Nrdot=-4;

Xu=0;
Yv=0;
Zw=0;
Kp=0;
Mq=0;
Nr=0;

Xuu=-34.55;
Yvv=-104.40;
Zww=-146.50;
Kpp=-0.68;
Mqq=-5.34;
Nrr=-3.07;


%govering equation is :M*Vdot+C*V+D*V+G=TAVc+TAVdisturbance
%TAVc is control force and moment in thruster and TAVdisturbance is disturbance force and moment
%M=Mrb+Madd is mass or inertia matrix

Mrb=[m 0 0 0 m*zg -m*yg;0 m 0 -m*zg 0 m*xg;0 0 m m*yg -m*xg 0;0 -m*zg m*yg Ixx -Ixy -Ixz ;m*zg 0 -m*xg -Ixy Iyy -Iyz;-m*yg m*xg 0 -Ixz -Iyz Izz];
Madd=-[Xudot Xvdot Xwdot Xpdot Xqdot Xrdot;Yudot Yvdot Ywdot Ypdot Yqdot Yrdot;Zudot Zvdot Zwdot Zpdot Zqdot Zrdot;Kudot Kvdot Kwdot Kpdot Kqdot Krdot;Mudot Mvdot Mwdot Mpdot Mqdot Mrdot;Nudot Nvdot Nwdot Npdot Nqdot Nrdot];
M=Mrb+Madd;
 

M;


%C=Crb+Cadd is coriolis matrix

a1=Xudot*u+ Xvdot*v +Xwdot*w+ Xpdot*p+ Xqdot*q+ Xrdot*r;
a2=Xudot*u+Yvdot*v+ Ywdot*w+ Ypdot*p+ Yqdot*q+ Yrdot*r;
a3=Xudot*u+Yvdot*v+ Zwdot*w+ Zpdot*p+ Zqdot*q+ Zrdot*r;
b1=Xudot*u+ Yvdot*v+ Zwdot*w+ Kpdot*p+ Kqdot*q+ Krdot*r;
b2=Xudot*u+ Yvdot*v+ Zwdot*w+ Kpdot*p+ Mqdot*q+ Mrdot*r;
b3=Xudot*u+ Yvdot*v+ Zwdot*w+ Kpdot*p+ Mqdot*q+ Nrdot*r;
Cadd=[0 0 0 0 -a3 a2;0 0 0 a3 0 -a1;0 0 0 -a2 a1 0;0 -a3 a2 0 -b3 b2;a3 0 -a1 b3 0 -b1;-a2 a1 0 -b2 b1 0];
C11=zeros(3,3);
C12=[m*(yg*q+zg*r) -m*(xg*q-w) -m*(xg*r+v);-m*(yg*q+w) m*(zg*r+xg*p) -m*(yg*r-u);-m*(zg*p-v) -m*(zg*q+u) m*(xg*p +yg*q)];
C22=[0 -Iyz*q-Ixz*p+Izz*r Iyz*r+Ixy*p-Iyy*q;Iyz*q+Ixz*p-Izz*r 0 -Ixz*r-Ixy*q+Ixx*p; -Iyz*r-Ixy*p+Iyy*q  Ixz*r+Ixy*q-Ixx*p 0];
Crb=[C11 C12;-C12' C22];
C=Crb+Cadd;





%D=D(linear drag coefficient)+D(quadratic drag coefficient) is hydrodynamic
%damping matrix 
%in this symolation  linear drag coefficientes are negligible

Dlinear=-[Xu 0 0 0 0 0;0 Yv 0 0 0 0;0 0 Zw 0 0 0 ;0 0 0 Kp 0 0 ;0 0 0 0 Mq 0;0 0 0 0 0 Nr];
Dquadratic=-[Xuu*abs(u) 0 0 0 0 0;0 Yvv*abs(v) 0 0 0 0;0 0 Zww*abs(w) 0 0 0 ;0 0 0 Kpp*abs(p) 0 0 ;0 0 0 0 Mqq*abs(q) 0;0 0 0 0 0 Nrr*abs(r)];
D=Dlinear+Dquadratic;


%G is gravity and bouancy vector that can be negligible
%because HM-AUV has natural bouancy and center of bouancy and  mass are coincide


%physical parameters of the vehicle
%w=yl=yr;
width=0.45;
%l=xt+xl=xt+xr;
l=0.885;
xl=0.135;
xr=0.135;
xt=0.75;

%defining the control force and moment of the thrusters as the inverse
%jacobian matrix of the error (e=current-desired position)
TAVcontrol=Jinv*e;

%according to the configuration of the vehicle, only the right and left
%thrusters contribute to x component of the force, all the three thrusters
%contribute to the z component of the force and only the tail thruster
%contributes to the y component of the force

fxthruster=TAVcontrol(1)/2;
fythruster=TAVcontrol(2);
fzthruster=TAVcontrol(3)/3;

%the added moment of thrusters in each direction should add up to zero and
%from this, the equations of added roll, pitch and yaw were drived as
%follows

fzaddroll2=TAVcontrol(4)/width;
fzaddroll1=TAVcontrol(4)/width;

fzaddpitch3=TAVcontrol(5)/l;
fzaddpitch2=TAVcontrol(5)/2*l;
fzaddpitch1=TAVcontrol(5)/2*l;

fxaddyaw2=TAVcontrol(6)/2*xl;
fxaddyaw1=TAVcontrol(6)/2*xr;


fxaddsway2=TAVcontrol(2)*xt/2*xl;
fxaddsway1=TAVcontrol(2)*xt/2*xr;

%due to the specific symmetry of the vehicle, the x, y, and z componets of
%the force generated by each thruster were drived
fzthruster1=fzthruster-fzaddroll1+fzaddpitch1;
fzthruster2=fzthruster+fzaddroll2+fzaddpitch2;
fzthruster3=fzthruster-fzaddpitch3;

fxthruster1=fxthruster+fxaddyaw1-fxaddsway1;
fxthruster2=fxthruster-fxaddyaw2+fxaddsway2;

fythruster3=fythruster;



%the magnitude of the total force of each thruster 
f1=sqrt(fxthruster1^2+fzthruster1^2);
f2=sqrt(fxthruster2^2+fzthruster2^2);
f3=sqrt(fythruster3^2+fzthruster3^2);

%govering equation is :M*Vdot+C*V+D*V+G=TAVcontrol and solving for Vdot aka
%acceleration which will be in need for the other blocks
Mfactor=inv(M)*TAVcontrol;
Cfactor=inv(M)*C*[u;v;w;p;q;r];
Dfactor=inv(M)*D*[u;v;w;p;q;r];

accelaration=Mfactor-Cfactor-Dfactor-inv(M)*tavdisturbance;

%calculating the theta angle for each thruster (rad)



thruster1teta=atan2(fzthruster1,fxthruster1);
thruster2teta=atan2(fzthruster2,fxthruster2);
thruster3teta=atan2(fzthruster3,fythruster3);





F=[f1;f2;f3];
